simulink model "sysTimeDemo"  (Simulink 7.9)
settings: Solver=ode45  StartTime=0.0  StopTime=inf  RelTol=1e-3
libraries: rtwinlib x1, LibreriaSimulinkINAUT x1
settings Model: Creator=dds  LastModifiedBy=aurora
settings DataIOCC: SignalLoggingSaveFormat=Dataset
settings OptimizationCC: ExpressionDepthLimit=128
settings DebuggingCC: UnderspecifiedInitializationDetection=Simplified  MergeDetectMultiDrivingBlocksExec=error  MultiTaskDSMMsg=warning  MultiTaskCondExecSysMsg=none  StateNameClashWarn=none  StrictBusMsg=None
settings RTWCC: IncludeERTFirstTime=on
settings CodeAppCC: CustomSymbolStrType=$N$R$M_T
settings GRTTargetCC: CodeReplacementLibrary=None  CPPClassGenCompliant=on

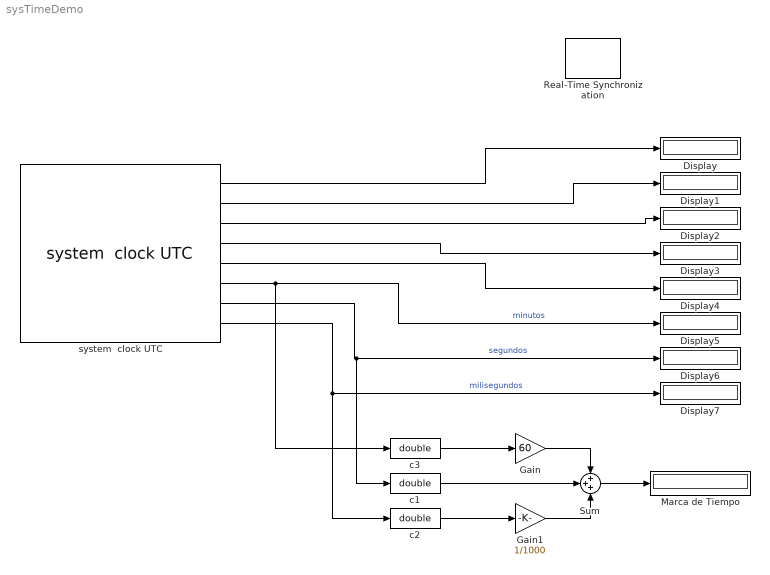
== system sysTimeDemo ==
  Display{,1..7} (8 alike) : Display
  Gain : Gain  Gain=60
  Gain1 : Gain  Gain=1/1000
  Marca de Tiempo : Display
  Real-Time Synchronization : rtwinlib/Real-Time Synchronization  SampleTime=0.1  MaxMissedTicks=10  ShowMissedTicks=off  YieldWhenWaiting=off
  Sum : Sum  Inputs=+++
  c1 : DataTypeConversion  OutDataTypeStr=double
  c2 : DataTypeConversion  OutDataTypeStr=double
  c3 : DataTypeConversion  OutDataTypeStr=double
  system  clock UTC : LibreriaSimulinkINAUT/system  clock UTC
  wires:
  system  clock UTC/1 -> Display/1
  system  clock UTC/2 -> Display1/1
  system  clock UTC/3 -> Display2/1
  system  clock UTC/4 -> Display3/1
  system  clock UTC/5 -> Display4/1
  system  clock UTC/6 -> c3/1, Display5/1  "minutos"
  system  clock UTC/7 -> Display6/1, c1/1  "segundos"
  system  clock UTC/8 -> c2/1, Display7/1  "milisegundos"
  Gain1/1 -> Sum/3
  Gain/1 -> Sum/1
  Sum/1 -> Marca de Tiempo/1
  c1/1 -> Sum/2
  c2/1 -> Gain1/1
  c3/1 -> Gain/1
